simulink model "stp1_4sym"  (R2022b)
settings: Solver=VariableStepAuto  StartTime=0.0  StopTime=10.0  RelTol=1e-3
values from neighbouring files (symbols this model uses):
  L = acker(A', C', [s0 s0 s0])    [stp1.m]
settings Model: Creator=zalew  LastModifiedBy=zalew

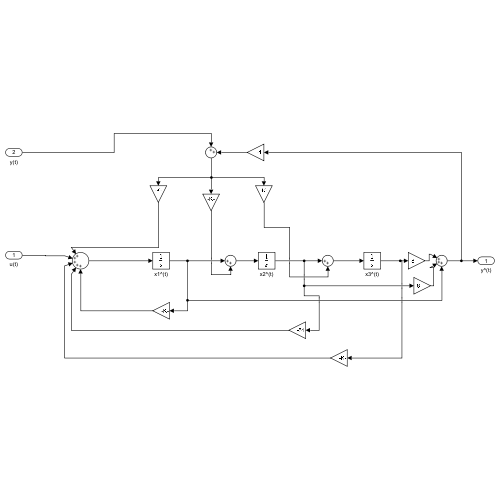
[thumbnail: Simulink's stored preview of the top-level diagram]
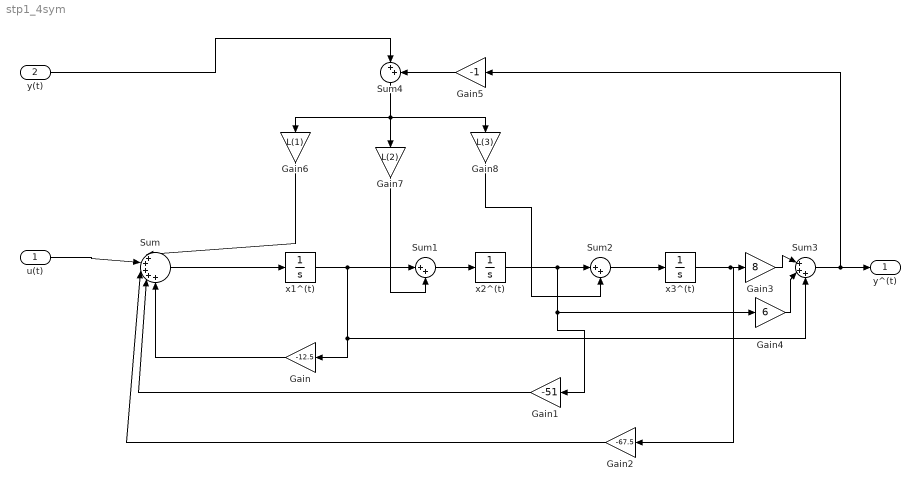
== system stp1_4sym ==
  u(t) : Inport
  y(t) : Inport  Port=2
  Gain : Gain  Gain=-12.5
  Gain1 : Gain  Gain=-51
  Gain2 : Gain  Gain=-67.5
  Gain3 : Gain  Gain=8
  Gain4 : Gain  Gain=6
  Gain5 : Gain  Gain=-1
  Gain6 : Gain  Gain=L(1)
  Gain7 : Gain  Gain=L(2)
  Gain8 : Gain  Gain=L(3)
  Sum : Sum  Inputs=|+++++
  Sum1 : Sum  Inputs=|++
  Sum2 : Sum  Inputs=|++
  Sum3 : Sum  Inputs=|+++
  Sum4 : Sum  Inputs=|++
  x1^(t) : Integrator
  x2^(t) : Integrator
  x3^(t) : Integrator
  y^(t) : Outport
  wires:
  u(t)/1 -> Sum/2
  Sum/1 -> x1^(t)/1
  x1^(t)/1 -> Sum3/3, Gain/1, Sum1/1
  Sum1/1 -> x2^(t)/1
  x2^(t)/1 -> Gain4/1, Gain1/1, Sum2/1
  Sum2/1 -> x3^(t)/1
  x3^(t)/1 -> Gain2/1, Gain3/1
  Sum3/1 -> Gain5/1, y^(t)/1
  y(t)/1 -> Sum4/1
  Gain/1 -> Sum/5
  Gain1/1 -> Sum/4
  Gain2/1 -> Sum/3
  Gain3/1 -> Sum3/1
  Gain4/1 -> Sum3/2
  Gain5/1 -> Sum4/2
  Sum4/1 -> Gain8/1, Gain7/1, Gain6/1
  Gain6/1 -> Sum/1
  Gain7/1 -> Sum1/2
  Gain8/1 -> Sum2/2
